simulink model "linear123"  (Simulink 7.8)
settings: Solver=ode45  StartTime=0.0  StopTime=10.0  RelTol=1e-3
libraries: powerlib x7
settings Model: Creator=sundeep  LastModifiedBy=sundeep

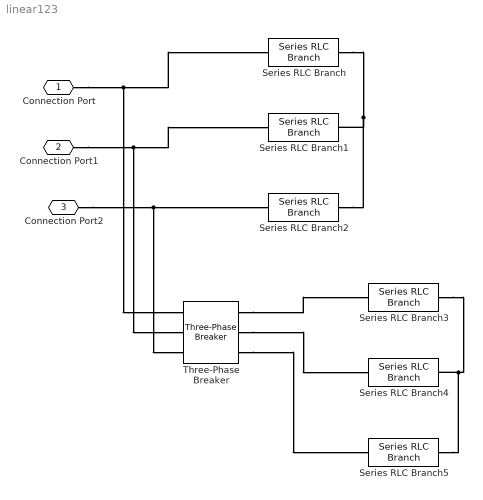
== system linear123 ==
  Series RLC Branch{,1..5} (6 alike) : powerlib/Elements/Series RLC Branch  LConnTagsString=__new0  RConnTagsString=__new0  BranchType=R  Resistance=1  Inductance=1e-3  SetiL0=off  InitialCurrent=0  Capacitance=1e-6  Setx0=off  InitialVoltage=0  Measurements=None
  Three-Phase Breaker : powerlib/Elements/Three-Phase Breaker  InitialState=open  SwitchA=on  SwitchB=on  SwitchC=on  SwitchTimes="[4/60  10/60]"  External=off  BreakerResistance=0.001  SnubberResistance=1e6  SnubberCapacitance=inf  Measurements=None
  Connection Port : PMIOPort  Port=1  Side=Left
  Connection Port1 : PMIOPort  Port=2  Side=Right
  Connection Port2 : PMIOPort  Port=3  Side=Left
  connections:
  Connection Port/RConn1 -- Series RLC Branch/LConn1 -- Three-Phase Breaker/LConn1
  Connection Port1/RConn1 -- Series RLC Branch1/LConn1 -- Three-Phase Breaker/LConn2
  Connection Port2/RConn1 -- Series RLC Branch2/LConn1 -- Three-Phase Breaker/LConn3
  Three-Phase Breaker/RConn1 -- Series RLC Branch3/LConn1
  Three-Phase Breaker/RConn2 -- Series RLC Branch4/LConn1
  Three-Phase Breaker/RConn3 -- Series RLC Branch5/LConn1
  Series RLC Branch/RConn1 -- Series RLC Branch1/RConn1 -- Series RLC Branch2/RConn1
  Series RLC Branch3/RConn1 -- Series RLC Branch4/RConn1 -- Series RLC Branch5/RConn1
